simulink model "can_simple_block_bu11143"  (R2016b)
settings: Solver=FixedStepDiscrete  StartTime=0.0  StopTime=1000  FixedStep=0.2  RelTol=1e-3  EnableMultiTasking=on
undefined symbols (not defined in the file or in its folder): A, A10, A14, B, B11, B12, B13, B8, C, CS0, CS1, D, D11, D4, F3, F4, G, G3, G4, H3, H4, K17, K4, L3, N16, PA11, PA12, PD0, PE14, PE15, R10, R14, R17, SCK, SIN, SOUT, T14
libraries: rappid_564xl_ec_toolbox x59
(part 5 of 6)

== matlab function can_simple_block_bu11143/DataDumpFast1/RawData to StoreData15 ==
  data: StrCell input; CellV_1_104 data_store_memory; VTDataCAN_8b output uint8
function VTDataCAN_8b = fcn(StrCell)
global CellV_1_104;
onemask8 = uint16(hex2dec('00FF'));
onemask8_8sft = uint16(hex2dec('FF00'));
onemask8_56sft = uint64(hex2dec('FF'));
% yl = uint8(bitand(u,onemask8));
% yh = uint8(bitsra(bitand(u,onemask8_8sft),8));
% bitshift(remainder,8)  shift left
% bitsra(remainder,8)  shift right



VTDataCAN_8b =  uint8(zeros(1,8));
VTDataCAN_64b =  uint64(zeros(1,1));
VTDataCAN_4data =  uint8(zeros(1,4));

% VTDataCAN_4data(1) = fix(CellV_1_104(StrCell*4-3)/4);
% VTDataCAN_4data(2) = fix(CellV_1_104(StrCell*4-2)/4);
% VTDataCAN_4data(3) = fix(CellV_1_104(StrCell*4-1)/4);
% VTDataCAN_4data(4) = fix(CellV_1_104(StrCell*4-0)/4);

Bid = StrCell;
VTDataCAN_64b = uint64( Bid ) + ...
                            uint64( bitshift(uint64(CellV_1_104(StrCell*4-3)/4),8 ) ) + ...
                            uint64( bitshift(uint64(CellV_1_104(StrCell*4-2)/4),8+14 ))  + ...
                            uint64( bitshift(uint64(CellV_1_104(StrCell*4-1)/4),8+14+14)  )  + ...
                            uint64( bitshift(uint64(CellV_1_104(StrCell*4-0)/4),8+14+14+14) ) ;

VTDataCAN_8b(1) = uint8( bitand(VTDataCAN_64b,onemask8_56sft) );
VTDataCAN_8b(2) = uint8( bitand(bitsra(VTDataCAN_64b,8*1),onemask8_56sft) );
VTDataCAN_8b(3) = uint8( bitand(bitsra(VTDataCAN_64b,8*2),onemask8_56sft) );
VTDataCAN_8b(4) = uint8( bitand(bitsra(VTDataCAN_64b,8*3),onemask8_56sft) );
VTDataCAN_8b(5) = uint8( bitand(bitsra(VTDataCAN_64b,8*4),onemask8_56sft) );
VTDataCAN_8b(6) = uint8( bitand(bitsra(VTDataCAN_64b,8*5),onemask8_56sft) );
VTDataCAN_8b(7) = uint8( bitand(bitsra(VTDataCAN_64b,8*6),onemask8_56sft) );
VTDataCAN_8b(8) = uint8( bitand(bitsra(VTDataCAN_64b,8*7),onemask8_56sft) );

% VTDataCAN_8b(1) = Bid;
% VTDataCAN_8b(2) = VTDataCAN_4data(1)/(2^8);
% VTDataCAN_8b(3) = 4*fix(mod(CellV_1_104(StrCell*4-3),2^8)/4);
% VTDataCAN_8b(3) = VTDataCAN_8b(3) + CellV_1_104(StrCell*4-2)/(2^14);
% VTDataCAN_8b(4) = mod(CellV_1_104(StrCell*4-2),2^14) / (2^8);
% VTDataCAN_8b(5) =  * fix(mod(CellV_1_104(StrCell*4-2),2^6));

4*fix(CellV_1_104(StrCell*4-3)/4);


% VTDataCAN_8b(1) =         CellV_1_104(StrCell*4-3)/256;
% VTDataCAN_8b(2) = mod(CellV_1_104(StrCell*4-3),256);
% VTDataCAN_8b(3) =         CellV_1_104(StrCell*4-2)/256;
% VTDataCAN_8b(4) = mod(CellV_1_104(StrCell*4-2),256);
% VTDataCAN_8b(5) =         CellV_1_104(StrCell*4-1)/256;
% VTDataCAN_8b(6) = mod(CellV_1_104(StrCell*4-1),256);
% VTDataCAN_8b(7) =         CellV_1_104(StrCell*4   )/256;
% VTDataCAN_8b(8) = mod(CellV_1_104(StrCell*4   ),256);

% VTDataCAN_8b(1) =         CellV_1_104(1)/256;
% VTDataCAN_8b(2) = mod(CellV_1_104(1),256);
% VTDataCAN_8b(3) =         CellV_1_104(2)/256;
% VTDataCAN_8b(4) = mod(CellV_1_104(2),256);
% VTDataCAN_8b(5) =         CellV_1_104(9)/256;
% VTDataCAN_8b(6) = mod(CellV_1_104(9),256);
% VTDataCAN_8b(7) =         CellV_1_104(10)/256;
% VTDataCAN_8b(8) = mod(CellV_1_104(10),256);

% VTDataCAN_8b(1) =         uint16(30000)/256;
% VTDataCAN_8b(2) = mod(uint16(30000),256);
% VTDataCAN_8b(3) =         uint16(35000)/256;
% VTDataCAN_8b(4) = mod(uint16(35000),256);
% VTDataCAN_8b(5) =         uint16(33000)/256;
% VTDataCAN_8b(6) = mod(uint16(33000),256);
% VTDataCAN_8b(7) =         uint16(20000)/256;
% VTDataCAN_8b(8) = mod(uint16(20000),256);


end








% CellV_1_104(1) = uint16(1);

% SPIDataStore = uint16(zeros(1,21));
% DataFault =  zeros(1,7);
%
% for i=1:7
%   SPIDataStore(i*3-2) = SPIData(i*8-7)+SPIData(i*8-6)*256;
%   SPIDataStore(i*3-1) = SPIData(i*8-5)+SPIData(i*8-4)*256;
%   SPIDataStore(i*3   ) = SPIData(i*8-3)+SPIData(i*8-2)*256;
%   if (PecChk(i*2-1) == SPIData(i*8-1)) && (PecChk(i*2) == SPIData(i*8))
%     DataFault(i) = 1;
%   else
%     DataFault(i) = 0;
%   end
% end



% onemask8 = uint16(hex2dec('00FF'));
% onemask8_8sft = uint16(hex2dec('FF00'));
% onemask88 = uint8(hex2dec('FF'));
% onemask16 = uint16(hex2dec('FFFF'));
%
% % data_test = zeros(1,2);
% remainder = uint16(16);
%
% for i=1:len
%     ii = uint16(i);
% %     data_test(1,i) = data(ii);
% %     address = 2;
%     address = bitand( ...
%         bitxor( ...
%         uint8(bitsra(remainder,7)),data(ii) ), ...
%         onemask88);
%     remainder = bitxor(bitshift(remainder,8,'uint16'),pec15Table(address+1));
% end
% pec15 = uint16(bitand(bitshift(remainder,1,'uint16'),onemask16));
% pec0 = uint8(bitand(pec15,onemask8));
% pec1 = uint8(bitsra(bitand(pec15,onemask8_8sft),8));

== matlab function can_simple_block_bu11143/DataDumpFast1/RawData to StoreData16 ==
  data: StrCell input; CellV_1_104 data_store_memory; VTDataCAN_8b output uint8
function VTDataCAN_8b = fcn(StrCell)
global CellV_1_104;
onemask8 = uint16(hex2dec('00FF'));
onemask8_8sft = uint16(hex2dec('FF00'));
onemask8_56sft = uint64(hex2dec('FF'));
% yl = uint8(bitand(u,onemask8));
% yh = uint8(bitsra(bitand(u,onemask8_8sft),8));
% bitshift(remainder,8)  shift left
% bitsra(remainder,8)  shift right



VTDataCAN_8b =  uint8(zeros(1,8));
VTDataCAN_64b =  uint64(zeros(1,1));
VTDataCAN_4data =  uint8(zeros(1,4));

% VTDataCAN_4data(1) = fix(CellV_1_104(StrCell*4-3)/4);
% VTDataCAN_4data(2) = fix(CellV_1_104(StrCell*4-2)/4);
% VTDataCAN_4data(3) = fix(CellV_1_104(StrCell*4-1)/4);
% VTDataCAN_4data(4) = fix(CellV_1_104(StrCell*4-0)/4);

Bid = StrCell;
VTDataCAN_64b = uint64( Bid ) + ...
                            uint64( bitshift(uint64(CellV_1_104(StrCell*4-3)/4),8 ) ) + ...
                            uint64( bitshift(uint64(CellV_1_104(StrCell*4-2)/4),8+14 ))  + ...
                            uint64( bitshift(uint64(CellV_1_104(StrCell*4-1)/4),8+14+14)  )  + ...
                            uint64( bitshift(uint64(CellV_1_104(StrCell*4-0)/4),8+14+14+14) ) ;

VTDataCAN_8b(1) = uint8( bitand(VTDataCAN_64b,onemask8_56sft) );
VTDataCAN_8b(2) = uint8( bitand(bitsra(VTDataCAN_64b,8*1),onemask8_56sft) );
VTDataCAN_8b(3) = uint8( bitand(bitsra(VTDataCAN_64b,8*2),onemask8_56sft) );
VTDataCAN_8b(4) = uint8( bitand(bitsra(VTDataCAN_64b,8*3),onemask8_56sft) );
VTDataCAN_8b(5) = uint8( bitand(bitsra(VTDataCAN_64b,8*4),onemask8_56sft) );
VTDataCAN_8b(6) = uint8( bitand(bitsra(VTDataCAN_64b,8*5),onemask8_56sft) );
VTDataCAN_8b(7) = uint8( bitand(bitsra(VTDataCAN_64b,8*6),onemask8_56sft) );
VTDataCAN_8b(8) = uint8( bitand(bitsra(VTDataCAN_64b,8*7),onemask8_56sft) );

% VTDataCAN_8b(1) = Bid;
% VTDataCAN_8b(2) = VTDataCAN_4data(1)/(2^8);
% VTDataCAN_8b(3) = 4*fix(mod(CellV_1_104(StrCell*4-3),2^8)/4);
% VTDataCAN_8b(3) = VTDataCAN_8b(3) + CellV_1_104(StrCell*4-2)/(2^14);
% VTDataCAN_8b(4) = mod(CellV_1_104(StrCell*4-2),2^14) / (2^8);
% VTDataCAN_8b(5) =  * fix(mod(CellV_1_104(StrCell*4-2),2^6));

4*fix(CellV_1_104(StrCell*4-3)/4);


% VTDataCAN_8b(1) =         CellV_1_104(StrCell*4-3)/256;
% VTDataCAN_8b(2) = mod(CellV_1_104(StrCell*4-3),256);
% VTDataCAN_8b(3) =         CellV_1_104(StrCell*4-2)/256;
% VTDataCAN_8b(4) = mod(CellV_1_104(StrCell*4-2),256);
% VTDataCAN_8b(5) =         CellV_1_104(StrCell*4-1)/256;
% VTDataCAN_8b(6) = mod(CellV_1_104(StrCell*4-1),256);
% VTDataCAN_8b(7) =         CellV_1_104(StrCell*4   )/256;
% VTDataCAN_8b(8) = mod(CellV_1_104(StrCell*4   ),256);

% VTDataCAN_8b(1) =         CellV_1_104(1)/256;
% VTDataCAN_8b(2) = mod(CellV_1_104(1),256);
% VTDataCAN_8b(3) =         CellV_1_104(2)/256;
% VTDataCAN_8b(4) = mod(CellV_1_104(2),256);
% VTDataCAN_8b(5) =         CellV_1_104(9)/256;
% VTDataCAN_8b(6) = mod(CellV_1_104(9),256);
% VTDataCAN_8b(7) =         CellV_1_104(10)/256;
% VTDataCAN_8b(8) = mod(CellV_1_104(10),256);

% VTDataCAN_8b(1) =         uint16(30000)/256;
% VTDataCAN_8b(2) = mod(uint16(30000),256);
% VTDataCAN_8b(3) =         uint16(35000)/256;
% VTDataCAN_8b(4) = mod(uint16(35000),256);
% VTDataCAN_8b(5) =         uint16(33000)/256;
% VTDataCAN_8b(6) = mod(uint16(33000),256);
% VTDataCAN_8b(7) =         uint16(20000)/256;
% VTDataCAN_8b(8) = mod(uint16(20000),256);


end








% CellV_1_104(1) = uint16(1);

% SPIDataStore = uint16(zeros(1,21));
% DataFault =  zeros(1,7);
%
% for i=1:7
%   SPIDataStore(i*3-2) = SPIData(i*8-7)+SPIData(i*8-6)*256;
%   SPIDataStore(i*3-1) = SPIData(i*8-5)+SPIData(i*8-4)*256;
%   SPIDataStore(i*3   ) = SPIData(i*8-3)+SPIData(i*8-2)*256;
%   if (PecChk(i*2-1) == SPIData(i*8-1)) && (PecChk(i*2) == SPIData(i*8))
%     DataFault(i) = 1;
%   else
%     DataFault(i) = 0;
%   end
% end



% onemask8 = uint16(hex2dec('00FF'));
% onemask8_8sft = uint16(hex2dec('FF00'));
% onemask88 = uint8(hex2dec('FF'));
% onemask16 = uint16(hex2dec('FFFF'));
%
% % data_test = zeros(1,2);
% remainder = uint16(16);
%
% for i=1:len
%     ii = uint16(i);
% %     data_test(1,i) = data(ii);
% %     address = 2;
%     address = bitand( ...
%         bitxor( ...
%         uint8(bitsra(remainder,7)),data(ii) ), ...
%         onemask88);
%     remainder = bitxor(bitshift(remainder,8,'uint16'),pec15Table(address+1));
% end
% pec15 = uint16(bitand(bitshift(remainder,1,'uint16'),onemask16));
% pec0 = uint8(bitand(pec15,onemask8));
% pec1 = uint8(bitsra(bitand(pec15,onemask8_8sft),8));

== stateflow chart can_simple_block_bu11143/DataDumpFast/Chart2 ==
  state A
    en: count  = count + 1;
    du: count = count + 1;
  state A1
    en: count = 1;
  (default) -> A : {count =0;}
  A1 -> A
  A -> A1 : [count >= count_in]
  data: count_in input; count output double [0..10000]

== matlab function can_simple_block_bu11143/DataDumpFast/RawData to StoreData1 ==
  data: StrCell input; CellGP_1_78 data_store_memory; VTDataCAN_8b output uint8
function VTDataCAN_8b = fcn(StrCell)

% global CellV_1_104;
global CellGP_1_78;
VTDataCAN_8b =  uint8(zeros(1,8));
% 
% StrCell_2 = fix((StrCell+1)/2);
% 
% if mod(StrCell,2)==1
% VTDataCAN_8b(1) =         CellGP_1_78(StrCell_2*6-5)/256;
% VTDataCAN_8b(2) = mod(CellGP_1_78(StrCell_2*6-5),256);
% VTDataCAN_8b(3) =         CellGP_1_78(StrCell_2*6-4)/256;
% VTDataCAN_8b(4) = mod(CellGP_1_78(StrCell_2*6-4),256);
% VTDataCAN_8b(5) =         CellGP_1_78(StrCell_2*6-3)/256;
% VTDataCAN_8b(6) = mod(CellGP_1_78(StrCell_2*6-3),256);
% VTDataCAN_8b(7) =         CellGP_1_78(StrCell_2*6-2 )/256;
% VTDataCAN_8b(8) = mod(CellGP_1_78(StrCell_2*6-2),256);
% else 
% VTDataCAN_8b(1) =         CellGP_1_78(StrCell_2*6-1 )/256;
% VTDataCAN_8b(2) = mod(CellGP_1_78(StrCell_2*6-1 ),256);
% VTDataCAN_8b(3) =         CellGP_1_78(StrCell_2*6-0 )/256;
% VTDataCAN_8b(4) = mod(CellGP_1_78(StrCell_2*6-0 ),256);
% end
onemask8 = uint16(hex2dec('00FF'));
onemask8_8sft = uint16(hex2dec('FF00'));
onemask8_56sft = uint64(hex2dec('FF'));
VTDataCAN_8b =  uint8(zeros(1,8));
VTDataCAN_64b =  uint64(zeros(1,1));
VTDataCAN_4data =  uint8(zeros(1,4));

Bid = StrCell;
VTDataCAN_64b = uint64( Bid ) + ...
                            uint64( bitshift(uint64(CellGP_1_78(StrCell*6-5)/64),8 ) ) + ...
                            uint64( bitshift(uint64(CellGP_1_78(StrCell*6-4)/64),8+10*1 ) )  + ...
                            uint64( bitshift(uint64(CellGP_1_78(StrCell*6-3)/64),8+10*2 ) )  + ...
                            uint64( bitshift(uint64(CellGP_1_78(StrCell*6-2)/64),8+10*3 ) ) + ...
                            uint64( bitshift(uint64(CellGP_1_78(StrCell*6-1)/64),8+10*4 ) ) + ...
                            uint64( bitshift(uint64(CellGP_1_78(StrCell*6-0)/1024),8+10*5 ) ) ;

VTDataCAN_8b(1) = uint8( bitand(VTDataCAN_64b,onemask8_56sft) );
VTDataCAN_8b(2) = uint8( bitand(bitsra(VTDataCAN_64b,8*1),onemask8_56sft) );
VTDataCAN_8b(3) = uint8( bitand(bitsra(VTDataCAN_64b,8*2),onemask8_56sft) );
VTDataCAN_8b(4) = uint8( bitand(bitsra(VTDataCAN_64b,8*3),onemask8_56sft) );
VTDataCAN_8b(5) = uint8( bitand(bitsra(VTDataCAN_64b,8*4),onemask8_56sft) );
VTDataCAN_8b(6) = uint8( bitand(bitsra(VTDataCAN_64b,8*5),onemask8_56sft) );
VTDataCAN_8b(7) = uint8( bitand(bitsra(VTDataCAN_64b,8*6),onemask8_56sft) );
VTDataCAN_8b(8) = uint8( bitand(bitsra(VTDataCAN_64b,8*7),onemask8_56sft) );


% VTDataCAN_8b(1) =         CellV_1_104(1)/256;
% VTDataCAN_8b(2) = mod(CellV_1_104(1),256);
% VTDataCAN_8b(3) =         CellV_1_104(2)/256;
% VTDataCAN_8b(4) = mod(CellV_1_104(2),256);
% VTDataCAN_8b(5) =         CellV_1_104(9)/256;
% VTDataCAN_8b(6) = mod(CellV_1_104(9),256);
% VTDataCAN_8b(7) =         CellV_1_104(10)/256;
% VTDataCAN_8b(8) = mod(CellV_1_104(10),256);

% VTDataCAN_8b(1) =         uint16(30000)/256;
% VTDataCAN_8b(2) = mod(uint16(30000),256);
% VTDataCAN_8b(3) =         uint16(35000)/256;
% VTDataCAN_8b(4) = mod(uint16(35000),256);
% VTDataCAN_8b(5) =         uint16(33000)/256;
% VTDataCAN_8b(6) = mod(uint16(33000),256);
% VTDataCAN_8b(7) =         uint16(20000)/256;
% VTDataCAN_8b(8) = mod(uint16(20000),256);


end








% CellV_1_104(1) = uint16(1);

% SPIDataStore = uint16(zeros(1,21));
% DataFault =  zeros(1,7);
%
% for i=1:7
%   SPIDataStore(i*3-2) = SPIData(i*8-7)+SPIData(i*8-6)*256;
%   SPIDataStore(i*3-1) = SPIData(i*8-5)+SPIData(i*8-4)*256;
%   SPIDataStore(i*3   ) = SPIData(i*8-3)+SPIData(i*8-2)*256;
%   if (PecChk(i*2-1) == SPIData(i*8-1)) && (PecChk(i*2) == SPIData(i*8))
%     DataFault(i) = 1;
%   else
%     DataFault(i) = 0;
%   end
% end



% onemask8 = uint16(hex2dec('00FF'));
% onemask8_8sft = uint16(hex2dec('FF00'));
% onemask88 = uint8(hex2dec('FF'));
% onemask16 = uint16(hex2dec('FFFF'));
%
% % data_test = zeros(1,2);
% remainder = uint16(16);
%
% for i=1:len
%     ii = uint16(i);
% %     data_test(1,i) = data(ii);
% %     address = 2;
%     address = bitand( ...
%         bitxor( ...
%         uint8(bitsra(remainder,7)),data(ii) ), ...
%         onemask88);
%     remainder = bitxor(bitshift(remainder,8,'uint16'),pec15Table(address+1));
% end
% pec15 = uint16(bitand(bitshift(remainder,1,'uint16'),onemask16));
% pec0 = uint8(bitand(pec15,onemask8));
% pec1 = uint8(bitsra(bitand(pec15,onemask8_8sft),8));

== matlab function can_simple_block_bu11143/DataDumpFast1/RawData to StoreData17 ==
  data: StrCell input; CellV_1_104 data_store_memory; VTDataCAN_8b output uint8
function VTDataCAN_8b = fcn(StrCell)
global CellV_1_104;
onemask8 = uint16(hex2dec('00FF'));
onemask8_8sft = uint16(hex2dec('FF00'));
onemask8_56sft = uint64(hex2dec('FF'));
% yl = uint8(bitand(u,onemask8));
% yh = uint8(bitsra(bitand(u,onemask8_8sft),8));
% bitshift(remainder,8)  shift left
% bitsra(remainder,8)  shift right



VTDataCAN_8b =  uint8(zeros(1,8));
VTDataCAN_64b =  uint64(zeros(1,1));
VTDataCAN_4data =  uint8(zeros(1,4));

% VTDataCAN_4data(1) = fix(CellV_1_104(StrCell*4-3)/4);
% VTDataCAN_4data(2) = fix(CellV_1_104(StrCell*4-2)/4);
% VTDataCAN_4data(3) = fix(CellV_1_104(StrCell*4-1)/4);
% VTDataCAN_4data(4) = fix(CellV_1_104(StrCell*4-0)/4);

Bid = StrCell;
VTDataCAN_64b = uint64( Bid ) + ...
                            uint64( bitshift(uint64(CellV_1_104(StrCell*4-3)/4),8 ) ) + ...
                            uint64( bitshift(uint64(CellV_1_104(StrCell*4-2)/4),8+14 ))  + ...
                            uint64( bitshift(uint64(CellV_1_104(StrCell*4-1)/4),8+14+14)  )  + ...
                            uint64( bitshift(uint64(CellV_1_104(StrCell*4-0)/4),8+14+14+14) ) ;

VTDataCAN_8b(1) = uint8( bitand(VTDataCAN_64b,onemask8_56sft) );
VTDataCAN_8b(2) = uint8( bitand(bitsra(VTDataCAN_64b,8*1),onemask8_56sft) );
VTDataCAN_8b(3) = uint8( bitand(bitsra(VTDataCAN_64b,8*2),onemask8_56sft) );
VTDataCAN_8b(4) = uint8( bitand(bitsra(VTDataCAN_64b,8*3),onemask8_56sft) );
VTDataCAN_8b(5) = uint8( bitand(bitsra(VTDataCAN_64b,8*4),onemask8_56sft) );
VTDataCAN_8b(6) = uint8( bitand(bitsra(VTDataCAN_64b,8*5),onemask8_56sft) );
VTDataCAN_8b(7) = uint8( bitand(bitsra(VTDataCAN_64b,8*6),onemask8_56sft) );
VTDataCAN_8b(8) = uint8( bitand(bitsra(VTDataCAN_64b,8*7),onemask8_56sft) );

% VTDataCAN_8b(1) = Bid;
% VTDataCAN_8b(2) = VTDataCAN_4data(1)/(2^8);
% VTDataCAN_8b(3) = 4*fix(mod(CellV_1_104(StrCell*4-3),2^8)/4);
% VTDataCAN_8b(3) = VTDataCAN_8b(3) + CellV_1_104(StrCell*4-2)/(2^14);
% VTDataCAN_8b(4) = mod(CellV_1_104(StrCell*4-2),2^14) / (2^8);
% VTDataCAN_8b(5) =  * fix(mod(CellV_1_104(StrCell*4-2),2^6));

4*fix(CellV_1_104(StrCell*4-3)/4);


% VTDataCAN_8b(1) =         CellV_1_104(StrCell*4-3)/256;
% VTDataCAN_8b(2) = mod(CellV_1_104(StrCell*4-3),256);
% VTDataCAN_8b(3) =         CellV_1_104(StrCell*4-2)/256;
% VTDataCAN_8b(4) = mod(CellV_1_104(StrCell*4-2),256);
% VTDataCAN_8b(5) =         CellV_1_104(StrCell*4-1)/256;
% VTDataCAN_8b(6) = mod(CellV_1_104(StrCell*4-1),256);
% VTDataCAN_8b(7) =         CellV_1_104(StrCell*4   )/256;
% VTDataCAN_8b(8) = mod(CellV_1_104(StrCell*4   ),256);

% VTDataCAN_8b(1) =         CellV_1_104(1)/256;
% VTDataCAN_8b(2) = mod(CellV_1_104(1),256);
% VTDataCAN_8b(3) =         CellV_1_104(2)/256;
% VTDataCAN_8b(4) = mod(CellV_1_104(2),256);
% VTDataCAN_8b(5) =         CellV_1_104(9)/256;
% VTDataCAN_8b(6) = mod(CellV_1_104(9),256);
% VTDataCAN_8b(7) =         CellV_1_104(10)/256;
% VTDataCAN_8b(8) = mod(CellV_1_104(10),256);

% VTDataCAN_8b(1) =         uint16(30000)/256;
% VTDataCAN_8b(2) = mod(uint16(30000),256);
% VTDataCAN_8b(3) =         uint16(35000)/256;
% VTDataCAN_8b(4) = mod(uint16(35000),256);
% VTDataCAN_8b(5) =         uint16(33000)/256;
% VTDataCAN_8b(6) = mod(uint16(33000),256);
% VTDataCAN_8b(7) =         uint16(20000)/256;
% VTDataCAN_8b(8) = mod(uint16(20000),256);


end








% CellV_1_104(1) = uint16(1);

% SPIDataStore = uint16(zeros(1,21));
% DataFault =  zeros(1,7);
%
% for i=1:7
%   SPIDataStore(i*3-2) = SPIData(i*8-7)+SPIData(i*8-6)*256;
%   SPIDataStore(i*3-1) = SPIData(i*8-5)+SPIData(i*8-4)*256;
%   SPIDataStore(i*3   ) = SPIData(i*8-3)+SPIData(i*8-2)*256;
%   if (PecChk(i*2-1) == SPIData(i*8-1)) && (PecChk(i*2) == SPIData(i*8))
%     DataFault(i) = 1;
%   else
%     DataFault(i) = 0;
%   end
% end



% onemask8 = uint16(hex2dec('00FF'));
% onemask8_8sft = uint16(hex2dec('FF00'));
% onemask88 = uint8(hex2dec('FF'));
% onemask16 = uint16(hex2dec('FFFF'));
%
% % data_test = zeros(1,2);
% remainder = uint16(16);
%
% for i=1:len
%     ii = uint16(i);
% %     data_test(1,i) = data(ii);
% %     address = 2;
%     address = bitand( ...
%         bitxor( ...
%         uint8(bitsra(remainder,7)),data(ii) ), ...
%         onemask88);
%     remainder = bitxor(bitshift(remainder,8,'uint16'),pec15Table(address+1));
% end
% pec15 = uint16(bitand(bitshift(remainder,1,'uint16'),onemask16));
% pec0 = uint8(bitand(pec15,onemask8));
% pec1 = uint8(bitsra(bitand(pec15,onemask8_8sft),8));

== matlab function can_simple_block_bu11143/DataDumpFast1/RawData to StoreData18 ==
  data: StrCell input; CellV_1_104 data_store_memory; VTDataCAN_8b output uint8
function VTDataCAN_8b = fcn(StrCell)
global CellV_1_104;
onemask8 = uint16(hex2dec('00FF'));
onemask8_8sft = uint16(hex2dec('FF00'));
onemask8_56sft = uint64(hex2dec('FF'));
% yl = uint8(bitand(u,onemask8));
% yh = uint8(bitsra(bitand(u,onemask8_8sft),8));
% bitshift(remainder,8)  shift left
% bitsra(remainder,8)  shift right



VTDataCAN_8b =  uint8(zeros(1,8));
VTDataCAN_64b =  uint64(zeros(1,1));
VTDataCAN_4data =  uint8(zeros(1,4));

% VTDataCAN_4data(1) = fix(CellV_1_104(StrCell*4-3)/4);
% VTDataCAN_4data(2) = fix(CellV_1_104(StrCell*4-2)/4);
% VTDataCAN_4data(3) = fix(CellV_1_104(StrCell*4-1)/4);
% VTDataCAN_4data(4) = fix(CellV_1_104(StrCell*4-0)/4);

Bid = StrCell;
VTDataCAN_64b = uint64( Bid ) + ...
                            uint64( bitshift(uint64(CellV_1_104(StrCell*4-3)/4),8 ) ) + ...
                            uint64( bitshift(uint64(CellV_1_104(StrCell*4-2)/4),8+14 ))  + ...
                            uint64( bitshift(uint64(CellV_1_104(StrCell*4-1)/4),8+14+14)  )  + ...
                            uint64( bitshift(uint64(CellV_1_104(StrCell*4-0)/4),8+14+14+14) ) ;

VTDataCAN_8b(1) = uint8( bitand(VTDataCAN_64b,onemask8_56sft) );
VTDataCAN_8b(2) = uint8( bitand(bitsra(VTDataCAN_64b,8*1),onemask8_56sft) );
VTDataCAN_8b(3) = uint8( bitand(bitsra(VTDataCAN_64b,8*2),onemask8_56sft) );
VTDataCAN_8b(4) = uint8( bitand(bitsra(VTDataCAN_64b,8*3),onemask8_56sft) );
VTDataCAN_8b(5) = uint8( bitand(bitsra(VTDataCAN_64b,8*4),onemask8_56sft) );
VTDataCAN_8b(6) = uint8( bitand(bitsra(VTDataCAN_64b,8*5),onemask8_56sft) );
VTDataCAN_8b(7) = uint8( bitand(bitsra(VTDataCAN_64b,8*6),onemask8_56sft) );
VTDataCAN_8b(8) = uint8( bitand(bitsra(VTDataCAN_64b,8*7),onemask8_56sft) );

% VTDataCAN_8b(1) = Bid;
% VTDataCAN_8b(2) = VTDataCAN_4data(1)/(2^8);
% VTDataCAN_8b(3) = 4*fix(mod(CellV_1_104(StrCell*4-3),2^8)/4);
% VTDataCAN_8b(3) = VTDataCAN_8b(3) + CellV_1_104(StrCell*4-2)/(2^14);
% VTDataCAN_8b(4) = mod(CellV_1_104(StrCell*4-2),2^14) / (2^8);
% VTDataCAN_8b(5) =  * fix(mod(CellV_1_104(StrCell*4-2),2^6));

4*fix(CellV_1_104(StrCell*4-3)/4);


% VTDataCAN_8b(1) =         CellV_1_104(StrCell*4-3)/256;
% VTDataCAN_8b(2) = mod(CellV_1_104(StrCell*4-3),256);
% VTDataCAN_8b(3) =         CellV_1_104(StrCell*4-2)/256;
% VTDataCAN_8b(4) = mod(CellV_1_104(StrCell*4-2),256);
% VTDataCAN_8b(5) =         CellV_1_104(StrCell*4-1)/256;
% VTDataCAN_8b(6) = mod(CellV_1_104(StrCell*4-1),256);
% VTDataCAN_8b(7) =         CellV_1_104(StrCell*4   )/256;
% VTDataCAN_8b(8) = mod(CellV_1_104(StrCell*4   ),256);

% VTDataCAN_8b(1) =         CellV_1_104(1)/256;
% VTDataCAN_8b(2) = mod(CellV_1_104(1),256);
% VTDataCAN_8b(3) =         CellV_1_104(2)/256;
% VTDataCAN_8b(4) = mod(CellV_1_104(2),256);
% VTDataCAN_8b(5) =         CellV_1_104(9)/256;
% VTDataCAN_8b(6) = mod(CellV_1_104(9),256);
% VTDataCAN_8b(7) =         CellV_1_104(10)/256;
% VTDataCAN_8b(8) = mod(CellV_1_104(10),256);

% VTDataCAN_8b(1) =         uint16(30000)/256;
% VTDataCAN_8b(2) = mod(uint16(30000),256);
% VTDataCAN_8b(3) =         uint16(35000)/256;
% VTDataCAN_8b(4) = mod(uint16(35000),256);
% VTDataCAN_8b(5) =         uint16(33000)/256;
% VTDataCAN_8b(6) = mod(uint16(33000),256);
% VTDataCAN_8b(7) =         uint16(20000)/256;
% VTDataCAN_8b(8) = mod(uint16(20000),256);


end








% CellV_1_104(1) = uint16(1);

% SPIDataStore = uint16(zeros(1,21));
% DataFault =  zeros(1,7);
%
% for i=1:7
%   SPIDataStore(i*3-2) = SPIData(i*8-7)+SPIData(i*8-6)*256;
%   SPIDataStore(i*3-1) = SPIData(i*8-5)+SPIData(i*8-4)*256;
%   SPIDataStore(i*3   ) = SPIData(i*8-3)+SPIData(i*8-2)*256;
%   if (PecChk(i*2-1) == SPIData(i*8-1)) && (PecChk(i*2) == SPIData(i*8))
%     DataFault(i) = 1;
%   else
%     DataFault(i) = 0;
%   end
% end



% onemask8 = uint16(hex2dec('00FF'));
% onemask8_8sft = uint16(hex2dec('FF00'));
% onemask88 = uint8(hex2dec('FF'));
% onemask16 = uint16(hex2dec('FFFF'));
%
% % data_test = zeros(1,2);
% remainder = uint16(16);
%
% for i=1:len
%     ii = uint16(i);
% %     data_test(1,i) = data(ii);
% %     address = 2;
%     address = bitand( ...
%         bitxor( ...
%         uint8(bitsra(remainder,7)),data(ii) ), ...
%         onemask88);
%     remainder = bitxor(bitshift(remainder,8,'uint16'),pec15Table(address+1));
% end
% pec15 = uint16(bitand(bitshift(remainder,1,'uint16'),onemask16));
% pec0 = uint8(bitand(pec15,onemask8));
% pec1 = uint8(bitsra(bitand(pec15,onemask8_8sft),8));

== matlab function can_simple_block_bu11143/DataDumpFast1/RawData to StoreData19 ==
  data: StrCell input; CellV_1_104 data_store_memory; VTDataCAN_8b output uint8
function VTDataCAN_8b = fcn(StrCell)
global CellV_1_104;
onemask8 = uint16(hex2dec('00FF'));
onemask8_8sft = uint16(hex2dec('FF00'));
onemask8_56sft = uint64(hex2dec('FF'));
% yl = uint8(bitand(u,onemask8));
% yh = uint8(bitsra(bitand(u,onemask8_8sft),8));
% bitshift(remainder,8)  shift left
% bitsra(remainder,8)  shift right



VTDataCAN_8b =  uint8(zeros(1,8));
VTDataCAN_64b =  uint64(zeros(1,1));
VTDataCAN_4data =  uint8(zeros(1,4));

% VTDataCAN_4data(1) = fix(CellV_1_104(StrCell*4-3)/4);
% VTDataCAN_4data(2) = fix(CellV_1_104(StrCell*4-2)/4);
% VTDataCAN_4data(3) = fix(CellV_1_104(StrCell*4-1)/4);
% VTDataCAN_4data(4) = fix(CellV_1_104(StrCell*4-0)/4);

Bid = StrCell;
VTDataCAN_64b = uint64( Bid ) + ...
                            uint64( bitshift(uint64(CellV_1_104(StrCell*4-3)/4),8 ) ) + ...
                            uint64( bitshift(uint64(CellV_1_104(StrCell*4-2)/4),8+14 ))  + ...
                            uint64( bitshift(uint64(CellV_1_104(StrCell*4-1)/4),8+14+14)  )  + ...
                            uint64( bitshift(uint64(CellV_1_104(StrCell*4-0)/4),8+14+14+14) ) ;

VTDataCAN_8b(1) = uint8( bitand(VTDataCAN_64b,onemask8_56sft) );
VTDataCAN_8b(2) = uint8( bitand(bitsra(VTDataCAN_64b,8*1),onemask8_56sft) );
VTDataCAN_8b(3) = uint8( bitand(bitsra(VTDataCAN_64b,8*2),onemask8_56sft) );
VTDataCAN_8b(4) = uint8( bitand(bitsra(VTDataCAN_64b,8*3),onemask8_56sft) );
VTDataCAN_8b(5) = uint8( bitand(bitsra(VTDataCAN_64b,8*4),onemask8_56sft) );
VTDataCAN_8b(6) = uint8( bitand(bitsra(VTDataCAN_64b,8*5),onemask8_56sft) );
VTDataCAN_8b(7) = uint8( bitand(bitsra(VTDataCAN_64b,8*6),onemask8_56sft) );
VTDataCAN_8b(8) = uint8( bitand(bitsra(VTDataCAN_64b,8*7),onemask8_56sft) );

% VTDataCAN_8b(1) = Bid;
% VTDataCAN_8b(2) = VTDataCAN_4data(1)/(2^8);
% VTDataCAN_8b(3) = 4*fix(mod(CellV_1_104(StrCell*4-3),2^8)/4);
% VTDataCAN_8b(3) = VTDataCAN_8b(3) + CellV_1_104(StrCell*4-2)/(2^14);
% VTDataCAN_8b(4) = mod(CellV_1_104(StrCell*4-2),2^14) / (2^8);
% VTDataCAN_8b(5) =  * fix(mod(CellV_1_104(StrCell*4-2),2^6));

4*fix(CellV_1_104(StrCell*4-3)/4);


% VTDataCAN_8b(1) =         CellV_1_104(StrCell*4-3)/256;
% VTDataCAN_8b(2) = mod(CellV_1_104(StrCell*4-3),256);
% VTDataCAN_8b(3) =         CellV_1_104(StrCell*4-2)/256;
% VTDataCAN_8b(4) = mod(CellV_1_104(StrCell*4-2),256);
% VTDataCAN_8b(5) =         CellV_1_104(StrCell*4-1)/256;
% VTDataCAN_8b(6) = mod(CellV_1_104(StrCell*4-1),256);
% VTDataCAN_8b(7) =         CellV_1_104(StrCell*4   )/256;
% VTDataCAN_8b(8) = mod(CellV_1_104(StrCell*4   ),256);

% VTDataCAN_8b(1) =         CellV_1_104(1)/256;
% VTDataCAN_8b(2) = mod(CellV_1_104(1),256);
% VTDataCAN_8b(3) =         CellV_1_104(2)/256;
% VTDataCAN_8b(4) = mod(CellV_1_104(2),256);
% VTDataCAN_8b(5) =         CellV_1_104(9)/256;
% VTDataCAN_8b(6) = mod(CellV_1_104(9),256);
% VTDataCAN_8b(7) =         CellV_1_104(10)/256;
% VTDataCAN_8b(8) = mod(CellV_1_104(10),256);

% VTDataCAN_8b(1) =         uint16(30000)/256;
% VTDataCAN_8b(2) = mod(uint16(30000),256);
% VTDataCAN_8b(3) =         uint16(35000)/256;
% VTDataCAN_8b(4) = mod(uint16(35000),256);
% VTDataCAN_8b(5) =         uint16(33000)/256;
% VTDataCAN_8b(6) = mod(uint16(33000),256);
% VTDataCAN_8b(7) =         uint16(20000)/256;
% VTDataCAN_8b(8) = mod(uint16(20000),256);


end








% CellV_1_104(1) = uint16(1);

% SPIDataStore = uint16(zeros(1,21));
% DataFault =  zeros(1,7);
%
% for i=1:7
%   SPIDataStore(i*3-2) = SPIData(i*8-7)+SPIData(i*8-6)*256;
%   SPIDataStore(i*3-1) = SPIData(i*8-5)+SPIData(i*8-4)*256;
%   SPIDataStore(i*3   ) = SPIData(i*8-3)+SPIData(i*8-2)*256;
%   if (PecChk(i*2-1) == SPIData(i*8-1)) && (PecChk(i*2) == SPIData(i*8))
%     DataFault(i) = 1;
%   else
%     DataFault(i) = 0;
%   end
% end



% onemask8 = uint16(hex2dec('00FF'));
% onemask8_8sft = uint16(hex2dec('FF00'));
% onemask88 = uint8(hex2dec('FF'));
% onemask16 = uint16(hex2dec('FFFF'));
%
% % data_test = zeros(1,2);
% remainder = uint16(16);
%
% for i=1:len
%     ii = uint16(i);
% %     data_test(1,i) = data(ii);
% %     address = 2;
%     address = bitand( ...
%         bitxor( ...
%         uint8(bitsra(remainder,7)),data(ii) ), ...
%         onemask88);
%     remainder = bitxor(bitshift(remainder,8,'uint16'),pec15Table(address+1));
% end
% pec15 = uint16(bitand(bitshift(remainder,1,'uint16'),onemask16));
% pec0 = uint8(bitand(pec15,onemask8));
% pec1 = uint8(bitsra(bitand(pec15,onemask8_8sft),8));

== matlab function can_simple_block_bu11143/DataDumpFast1/RawData to StoreData20 ==
  data: StrCell input; CellV_1_104 data_store_memory; VTDataCAN_8b output uint8
function VTDataCAN_8b = fcn(StrCell)
global CellV_1_104;
onemask8 = uint16(hex2dec('00FF'));
onemask8_8sft = uint16(hex2dec('FF00'));
onemask8_56sft = uint64(hex2dec('FF'));
% yl = uint8(bitand(u,onemask8));
% yh = uint8(bitsra(bitand(u,onemask8_8sft),8));
% bitshift(remainder,8)  shift left
% bitsra(remainder,8)  shift right



VTDataCAN_8b =  uint8(zeros(1,8));
VTDataCAN_64b =  uint64(zeros(1,1));
VTDataCAN_4data =  uint8(zeros(1,4));

% VTDataCAN_4data(1) = fix(CellV_1_104(StrCell*4-3)/4);
% VTDataCAN_4data(2) = fix(CellV_1_104(StrCell*4-2)/4);
% VTDataCAN_4data(3) = fix(CellV_1_104(StrCell*4-1)/4);
% VTDataCAN_4data(4) = fix(CellV_1_104(StrCell*4-0)/4);

Bid = StrCell;
VTDataCAN_64b = uint64( Bid ) + ...
                            uint64( bitshift(uint64(CellV_1_104(StrCell*4-3)/4),8 ) ) + ...
                            uint64( bitshift(uint64(CellV_1_104(StrCell*4-2)/4),8+14 ))  + ...
                            uint64( bitshift(uint64(CellV_1_104(StrCell*4-1)/4),8+14+14)  )  + ...
                            uint64( bitshift(uint64(CellV_1_104(StrCell*4-0)/4),8+14+14+14) ) ;

VTDataCAN_8b(1) = uint8( bitand(VTDataCAN_64b,onemask8_56sft) );
VTDataCAN_8b(2) = uint8( bitand(bitsra(VTDataCAN_64b,8*1),onemask8_56sft) );
VTDataCAN_8b(3) = uint8( bitand(bitsra(VTDataCAN_64b,8*2),onemask8_56sft) );
VTDataCAN_8b(4) = uint8( bitand(bitsra(VTDataCAN_64b,8*3),onemask8_56sft) );
VTDataCAN_8b(5) = uint8( bitand(bitsra(VTDataCAN_64b,8*4),onemask8_56sft) );
VTDataCAN_8b(6) = uint8( bitand(bitsra(VTDataCAN_64b,8*5),onemask8_56sft) );
VTDataCAN_8b(7) = uint8( bitand(bitsra(VTDataCAN_64b,8*6),onemask8_56sft) );
VTDataCAN_8b(8) = uint8( bitand(bitsra(VTDataCAN_64b,8*7),onemask8_56sft) );

% VTDataCAN_8b(1) = Bid;
% VTDataCAN_8b(2) = VTDataCAN_4data(1)/(2^8);
% VTDataCAN_8b(3) = 4*fix(mod(CellV_1_104(StrCell*4-3),2^8)/4);
% VTDataCAN_8b(3) = VTDataCAN_8b(3) + CellV_1_104(StrCell*4-2)/(2^14);
% VTDataCAN_8b(4) = mod(CellV_1_104(StrCell*4-2),2^14) / (2^8);
% VTDataCAN_8b(5) =  * fix(mod(CellV_1_104(StrCell*4-2),2^6));

4*fix(CellV_1_104(StrCell*4-3)/4);


% VTDataCAN_8b(1) =         CellV_1_104(StrCell*4-3)/256;
% VTDataCAN_8b(2) = mod(CellV_1_104(StrCell*4-3),256);
% VTDataCAN_8b(3) =         CellV_1_104(StrCell*4-2)/256;
% VTDataCAN_8b(4) = mod(CellV_1_104(StrCell*4-2),256);
% VTDataCAN_8b(5) =         CellV_1_104(StrCell*4-1)/256;
% VTDataCAN_8b(6) = mod(CellV_1_104(StrCell*4-1),256);
% VTDataCAN_8b(7) =         CellV_1_104(StrCell*4   )/256;
% VTDataCAN_8b(8) = mod(CellV_1_104(StrCell*4   ),256);

% VTDataCAN_8b(1) =         CellV_1_104(1)/256;
% VTDataCAN_8b(2) = mod(CellV_1_104(1),256);
% VTDataCAN_8b(3) =         CellV_1_104(2)/256;
% VTDataCAN_8b(4) = mod(CellV_1_104(2),256);
% VTDataCAN_8b(5) =         CellV_1_104(9)/256;
% VTDataCAN_8b(6) = mod(CellV_1_104(9),256);
% VTDataCAN_8b(7) =         CellV_1_104(10)/256;
% VTDataCAN_8b(8) = mod(CellV_1_104(10),256);

% VTDataCAN_8b(1) =         uint16(30000)/256;
% VTDataCAN_8b(2) = mod(uint16(30000),256);
% VTDataCAN_8b(3) =         uint16(35000)/256;
% VTDataCAN_8b(4) = mod(uint16(35000),256);
% VTDataCAN_8b(5) =         uint16(33000)/256;
% VTDataCAN_8b(6) = mod(uint16(33000),256);
% VTDataCAN_8b(7) =         uint16(20000)/256;
% VTDataCAN_8b(8) = mod(uint16(20000),256);


end








% CellV_1_104(1) = uint16(1);

% SPIDataStore = uint16(zeros(1,21));
% DataFault =  zeros(1,7);
%
% for i=1:7
%   SPIDataStore(i*3-2) = SPIData(i*8-7)+SPIData(i*8-6)*256;
%   SPIDataStore(i*3-1) = SPIData(i*8-5)+SPIData(i*8-4)*256;
%   SPIDataStore(i*3   ) = SPIData(i*8-3)+SPIData(i*8-2)*256;
%   if (PecChk(i*2-1) == SPIData(i*8-1)) && (PecChk(i*2) == SPIData(i*8))
%     DataFault(i) = 1;
%   else
%     DataFault(i) = 0;
%   end
% end



% onemask8 = uint16(hex2dec('00FF'));
% onemask8_8sft = uint16(hex2dec('FF00'));
% onemask88 = uint8(hex2dec('FF'));
% onemask16 = uint16(hex2dec('FFFF'));
%
% % data_test = zeros(1,2);
% remainder = uint16(16);
%
% for i=1:len
%     ii = uint16(i);
% %     data_test(1,i) = data(ii);
% %     address = 2;
%     address = bitand( ...
%         bitxor( ...
%         uint8(bitsra(remainder,7)),data(ii) ), ...
%         onemask88);
%     remainder = bitxor(bitshift(remainder,8,'uint16'),pec15Table(address+1));
% end
% pec15 = uint16(bitand(bitshift(remainder,1,'uint16'),onemask16));
% pec0 = uint8(bitand(pec15,onemask8));
% pec1 = uint8(bitsra(bitand(pec15,onemask8_8sft),8));

== matlab function can_simple_block_bu11143/DataDumpFast1/RawData to StoreData21 ==
  data: StrCell input; CellV_1_104 data_store_memory; VTDataCAN_8b output uint8
function VTDataCAN_8b = fcn(StrCell)
global CellV_1_104;
onemask8 = uint16(hex2dec('00FF'));
onemask8_8sft = uint16(hex2dec('FF00'));
onemask8_56sft = uint64(hex2dec('FF'));
% yl = uint8(bitand(u,onemask8));
% yh = uint8(bitsra(bitand(u,onemask8_8sft),8));
% bitshift(remainder,8)  shift left
% bitsra(remainder,8)  shift right



VTDataCAN_8b =  uint8(zeros(1,8));
VTDataCAN_64b =  uint64(zeros(1,1));
VTDataCAN_4data =  uint8(zeros(1,4));

% VTDataCAN_4data(1) = fix(CellV_1_104(StrCell*4-3)/4);
% VTDataCAN_4data(2) = fix(CellV_1_104(StrCell*4-2)/4);
% VTDataCAN_4data(3) = fix(CellV_1_104(StrCell*4-1)/4);
% VTDataCAN_4data(4) = fix(CellV_1_104(StrCell*4-0)/4);

Bid = StrCell;
VTDataCAN_64b = uint64( Bid ) + ...
                            uint64( bitshift(uint64(CellV_1_104(StrCell*4-3)/4),8 ) ) + ...
                            uint64( bitshift(uint64(CellV_1_104(StrCell*4-2)/4),8+14 ))  + ...
                            uint64( bitshift(uint64(CellV_1_104(StrCell*4-1)/4),8+14+14)  )  + ...
                            uint64( bitshift(uint64(CellV_1_104(StrCell*4-0)/4),8+14+14+14) ) ;

VTDataCAN_8b(1) = uint8( bitand(VTDataCAN_64b,onemask8_56sft) );
VTDataCAN_8b(2) = uint8( bitand(bitsra(VTDataCAN_64b,8*1),onemask8_56sft) );
VTDataCAN_8b(3) = uint8( bitand(bitsra(VTDataCAN_64b,8*2),onemask8_56sft) );
VTDataCAN_8b(4) = uint8( bitand(bitsra(VTDataCAN_64b,8*3),onemask8_56sft) );
VTDataCAN_8b(5) = uint8( bitand(bitsra(VTDataCAN_64b,8*4),onemask8_56sft) );
VTDataCAN_8b(6) = uint8( bitand(bitsra(VTDataCAN_64b,8*5),onemask8_56sft) );
VTDataCAN_8b(7) = uint8( bitand(bitsra(VTDataCAN_64b,8*6),onemask8_56sft) );
VTDataCAN_8b(8) = uint8( bitand(bitsra(VTDataCAN_64b,8*7),onemask8_56sft) );

% VTDataCAN_8b(1) = Bid;
% VTDataCAN_8b(2) = VTDataCAN_4data(1)/(2^8);
% VTDataCAN_8b(3) = 4*fix(mod(CellV_1_104(StrCell*4-3),2^8)/4);
% VTDataCAN_8b(3) = VTDataCAN_8b(3) + CellV_1_104(StrCell*4-2)/(2^14);
% VTDataCAN_8b(4) = mod(CellV_1_104(StrCell*4-2),2^14) / (2^8);
% VTDataCAN_8b(5) =  * fix(mod(CellV_1_104(StrCell*4-2),2^6));

4*fix(CellV_1_104(StrCell*4-3)/4);


% VTDataCAN_8b(1) =         CellV_1_104(StrCell*4-3)/256;
% VTDataCAN_8b(2) = mod(CellV_1_104(StrCell*4-3),256);
% VTDataCAN_8b(3) =         CellV_1_104(StrCell*4-2)/256;
% VTDataCAN_8b(4) = mod(CellV_1_104(StrCell*4-2),256);
% VTDataCAN_8b(5) =         CellV_1_104(StrCell*4-1)/256;
% VTDataCAN_8b(6) = mod(CellV_1_104(StrCell*4-1),256);
% VTDataCAN_8b(7) =         CellV_1_104(StrCell*4   )/256;
% VTDataCAN_8b(8) = mod(CellV_1_104(StrCell*4   ),256);

% VTDataCAN_8b(1) =         CellV_1_104(1)/256;
% VTDataCAN_8b(2) = mod(CellV_1_104(1),256);
% VTDataCAN_8b(3) =         CellV_1_104(2)/256;
% VTDataCAN_8b(4) = mod(CellV_1_104(2),256);
% VTDataCAN_8b(5) =         CellV_1_104(9)/256;
% VTDataCAN_8b(6) = mod(CellV_1_104(9),256);
% VTDataCAN_8b(7) =         CellV_1_104(10)/256;
% VTDataCAN_8b(8) = mod(CellV_1_104(10),256);

% VTDataCAN_8b(1) =         uint16(30000)/256;
% VTDataCAN_8b(2) = mod(uint16(30000),256);
% VTDataCAN_8b(3) =         uint16(35000)/256;
% VTDataCAN_8b(4) = mod(uint16(35000),256);
% VTDataCAN_8b(5) =         uint16(33000)/256;
% VTDataCAN_8b(6) = mod(uint16(33000),256);
% VTDataCAN_8b(7) =         uint16(20000)/256;
% VTDataCAN_8b(8) = mod(uint16(20000),256);


end








% CellV_1_104(1) = uint16(1);

% SPIDataStore = uint16(zeros(1,21));
% DataFault =  zeros(1,7);
%
% for i=1:7
%   SPIDataStore(i*3-2) = SPIData(i*8-7)+SPIData(i*8-6)*256;
%   SPIDataStore(i*3-1) = SPIData(i*8-5)+SPIData(i*8-4)*256;
%   SPIDataStore(i*3   ) = SPIData(i*8-3)+SPIData(i*8-2)*256;
%   if (PecChk(i*2-1) == SPIData(i*8-1)) && (PecChk(i*2) == SPIData(i*8))
%     DataFault(i) = 1;
%   else
%     DataFault(i) = 0;
%   end
% end



% onemask8 = uint16(hex2dec('00FF'));
% onemask8_8sft = uint16(hex2dec('FF00'));
% onemask88 = uint8(hex2dec('FF'));
% onemask16 = uint16(hex2dec('FFFF'));
%
% % data_test = zeros(1,2);
% remainder = uint16(16);
%
% for i=1:len
%     ii = uint16(i);
% %     data_test(1,i) = data(ii);
% %     address = 2;
%     address = bitand( ...
%         bitxor( ...
%         uint8(bitsra(remainder,7)),data(ii) ), ...
%         onemask88);
%     remainder = bitxor(bitshift(remainder,8,'uint16'),pec15Table(address+1));
% end
% pec15 = uint16(bitand(bitshift(remainder,1,'uint16'),onemask16));
% pec0 = uint8(bitand(pec15,onemask8));
% pec1 = uint8(bitsra(bitand(pec15,onemask8_8sft),8));

== matlab function can_simple_block_bu11143/DataDumpFast1/RawData to StoreData22 ==
  data: StrCell input; CellV_1_104 data_store_memory; VTDataCAN_8b output uint8
function VTDataCAN_8b = fcn(StrCell)
global CellV_1_104;
onemask8 = uint16(hex2dec('00FF'));
onemask8_8sft = uint16(hex2dec('FF00'));
onemask8_56sft = uint64(hex2dec('FF'));
% yl = uint8(bitand(u,onemask8));
% yh = uint8(bitsra(bitand(u,onemask8_8sft),8));
% bitshift(remainder,8)  shift left
% bitsra(remainder,8)  shift right



VTDataCAN_8b =  uint8(zeros(1,8));
VTDataCAN_64b =  uint64(zeros(1,1));
VTDataCAN_4data =  uint8(zeros(1,4));

% VTDataCAN_4data(1) = fix(CellV_1_104(StrCell*4-3)/4);
% VTDataCAN_4data(2) = fix(CellV_1_104(StrCell*4-2)/4);
% VTDataCAN_4data(3) = fix(CellV_1_104(StrCell*4-1)/4);
% VTDataCAN_4data(4) = fix(CellV_1_104(StrCell*4-0)/4);

Bid = StrCell;
VTDataCAN_64b = uint64( Bid ) + ...
                            uint64( bitshift(uint64(CellV_1_104(StrCell*4-3)/4),8 ) ) + ...
                            uint64( bitshift(uint64(CellV_1_104(StrCell*4-2)/4),8+14 ))  + ...
                            uint64( bitshift(uint64(CellV_1_104(StrCell*4-1)/4),8+14+14)  )  + ...
                            uint64( bitshift(uint64(CellV_1_104(StrCell*4-0)/4),8+14+14+14) ) ;

VTDataCAN_8b(1) = uint8( bitand(VTDataCAN_64b,onemask8_56sft) );
VTDataCAN_8b(2) = uint8( bitand(bitsra(VTDataCAN_64b,8*1),onemask8_56sft) );
VTDataCAN_8b(3) = uint8( bitand(bitsra(VTDataCAN_64b,8*2),onemask8_56sft) );
VTDataCAN_8b(4) = uint8( bitand(bitsra(VTDataCAN_64b,8*3),onemask8_56sft) );
VTDataCAN_8b(5) = uint8( bitand(bitsra(VTDataCAN_64b,8*4),onemask8_56sft) );
VTDataCAN_8b(6) = uint8( bitand(bitsra(VTDataCAN_64b,8*5),onemask8_56sft) );
VTDataCAN_8b(7) = uint8( bitand(bitsra(VTDataCAN_64b,8*6),onemask8_56sft) );
VTDataCAN_8b(8) = uint8( bitand(bitsra(VTDataCAN_64b,8*7),onemask8_56sft) );

% VTDataCAN_8b(1) = Bid;
% VTDataCAN_8b(2) = VTDataCAN_4data(1)/(2^8);
% VTDataCAN_8b(3) = 4*fix(mod(CellV_1_104(StrCell*4-3),2^8)/4);
% VTDataCAN_8b(3) = VTDataCAN_8b(3) + CellV_1_104(StrCell*4-2)/(2^14);
% VTDataCAN_8b(4) = mod(CellV_1_104(StrCell*4-2),2^14) / (2^8);
% VTDataCAN_8b(5) =  * fix(mod(CellV_1_104(StrCell*4-2),2^6));

4*fix(CellV_1_104(StrCell*4-3)/4);


% VTDataCAN_8b(1) =         CellV_1_104(StrCell*4-3)/256;
% VTDataCAN_8b(2) = mod(CellV_1_104(StrCell*4-3),256);
% VTDataCAN_8b(3) =         CellV_1_104(StrCell*4-2)/256;
% VTDataCAN_8b(4) = mod(CellV_1_104(StrCell*4-2),256);
% VTDataCAN_8b(5) =         CellV_1_104(StrCell*4-1)/256;
% VTDataCAN_8b(6) = mod(CellV_1_104(StrCell*4-1),256);
% VTDataCAN_8b(7) =         CellV_1_104(StrCell*4   )/256;
% VTDataCAN_8b(8) = mod(CellV_1_104(StrCell*4   ),256);

% VTDataCAN_8b(1) =         CellV_1_104(1)/256;
% VTDataCAN_8b(2) = mod(CellV_1_104(1),256);
% VTDataCAN_8b(3) =         CellV_1_104(2)/256;
% VTDataCAN_8b(4) = mod(CellV_1_104(2),256);
% VTDataCAN_8b(5) =         CellV_1_104(9)/256;
% VTDataCAN_8b(6) = mod(CellV_1_104(9),256);
% VTDataCAN_8b(7) =         CellV_1_104(10)/256;
% VTDataCAN_8b(8) = mod(CellV_1_104(10),256);

% VTDataCAN_8b(1) =         uint16(30000)/256;
% VTDataCAN_8b(2) = mod(uint16(30000),256);
% VTDataCAN_8b(3) =         uint16(35000)/256;
% VTDataCAN_8b(4) = mod(uint16(35000),256);
% VTDataCAN_8b(5) =         uint16(33000)/256;
% VTDataCAN_8b(6) = mod(uint16(33000),256);
% VTDataCAN_8b(7) =         uint16(20000)/256;
% VTDataCAN_8b(8) = mod(uint16(20000),256);


end








% CellV_1_104(1) = uint16(1);

% SPIDataStore = uint16(zeros(1,21));
% DataFault =  zeros(1,7);
%
% for i=1:7
%   SPIDataStore(i*3-2) = SPIData(i*8-7)+SPIData(i*8-6)*256;
%   SPIDataStore(i*3-1) = SPIData(i*8-5)+SPIData(i*8-4)*256;
%   SPIDataStore(i*3   ) = SPIData(i*8-3)+SPIData(i*8-2)*256;
%   if (PecChk(i*2-1) == SPIData(i*8-1)) && (PecChk(i*2) == SPIData(i*8))
%     DataFault(i) = 1;
%   else
%     DataFault(i) = 0;
%   end
% end



% onemask8 = uint16(hex2dec('00FF'));
% onemask8_8sft = uint16(hex2dec('FF00'));
% onemask88 = uint8(hex2dec('FF'));
% onemask16 = uint16(hex2dec('FFFF'));
%
% % data_test = zeros(1,2);
% remainder = uint16(16);
%
% for i=1:len
%     ii = uint16(i);
% %     data_test(1,i) = data(ii);
% %     address = 2;
%     address = bitand( ...
%         bitxor( ...
%         uint8(bitsra(remainder,7)),data(ii) ), ...
%         onemask88);
%     remainder = bitxor(bitshift(remainder,8,'uint16'),pec15Table(address+1));
% end
% pec15 = uint16(bitand(bitshift(remainder,1,'uint16'),onemask16));
% pec0 = uint8(bitand(pec15,onemask8));
% pec1 = uint8(bitsra(bitand(pec15,onemask8_8sft),8));

== matlab function can_simple_block_bu11143/DataDumpFast1/RawData to StoreData23 ==
  data: StrCell input; CellV_1_104 data_store_memory; VTDataCAN_8b output uint8
function VTDataCAN_8b = fcn(StrCell)
global CellV_1_104;
onemask8 = uint16(hex2dec('00FF'));
onemask8_8sft = uint16(hex2dec('FF00'));
onemask8_56sft = uint64(hex2dec('FF'));
% yl = uint8(bitand(u,onemask8));
% yh = uint8(bitsra(bitand(u,onemask8_8sft),8));
% bitshift(remainder,8)  shift left
% bitsra(remainder,8)  shift right



VTDataCAN_8b =  uint8(zeros(1,8));
VTDataCAN_64b =  uint64(zeros(1,1));
VTDataCAN_4data =  uint8(zeros(1,4));

% VTDataCAN_4data(1) = fix(CellV_1_104(StrCell*4-3)/4);
% VTDataCAN_4data(2) = fix(CellV_1_104(StrCell*4-2)/4);
% VTDataCAN_4data(3) = fix(CellV_1_104(StrCell*4-1)/4);
% VTDataCAN_4data(4) = fix(CellV_1_104(StrCell*4-0)/4);

Bid = StrCell;
VTDataCAN_64b = uint64( Bid ) + ...
                            uint64( bitshift(uint64(CellV_1_104(StrCell*4-3)/4),8 ) ) + ...
                            uint64( bitshift(uint64(CellV_1_104(StrCell*4-2)/4),8+14 ))  + ...
                            uint64( bitshift(uint64(CellV_1_104(StrCell*4-1)/4),8+14+14)  )  + ...
                            uint64( bitshift(uint64(CellV_1_104(StrCell*4-0)/4),8+14+14+14) ) ;

VTDataCAN_8b(1) = uint8( bitand(VTDataCAN_64b,onemask8_56sft) );
VTDataCAN_8b(2) = uint8( bitand(bitsra(VTDataCAN_64b,8*1),onemask8_56sft) );
VTDataCAN_8b(3) = uint8( bitand(bitsra(VTDataCAN_64b,8*2),onemask8_56sft) );
VTDataCAN_8b(4) = uint8( bitand(bitsra(VTDataCAN_64b,8*3),onemask8_56sft) );
VTDataCAN_8b(5) = uint8( bitand(bitsra(VTDataCAN_64b,8*4),onemask8_56sft) );
VTDataCAN_8b(6) = uint8( bitand(bitsra(VTDataCAN_64b,8*5),onemask8_56sft) );
VTDataCAN_8b(7) = uint8( bitand(bitsra(VTDataCAN_64b,8*6),onemask8_56sft) );
VTDataCAN_8b(8) = uint8( bitand(bitsra(VTDataCAN_64b,8*7),onemask8_56sft) );

% VTDataCAN_8b(1) = Bid;
% VTDataCAN_8b(2) = VTDataCAN_4data(1)/(2^8);
% VTDataCAN_8b(3) = 4*fix(mod(CellV_1_104(StrCell*4-3),2^8)/4);
% VTDataCAN_8b(3) = VTDataCAN_8b(3) + CellV_1_104(StrCell*4-2)/(2^14);
% VTDataCAN_8b(4) = mod(CellV_1_104(StrCell*4-2),2^14) / (2^8);
% VTDataCAN_8b(5) =  * fix(mod(CellV_1_104(StrCell*4-2),2^6));

4*fix(CellV_1_104(StrCell*4-3)/4);


% VTDataCAN_8b(1) =         CellV_1_104(StrCell*4-3)/256;
% VTDataCAN_8b(2) = mod(CellV_1_104(StrCell*4-3),256);
% VTDataCAN_8b(3) =         CellV_1_104(StrCell*4-2)/256;
% VTDataCAN_8b(4) = mod(CellV_1_104(StrCell*4-2),256);
% VTDataCAN_8b(5) =         CellV_1_104(StrCell*4-1)/256;
% VTDataCAN_8b(6) = mod(CellV_1_104(StrCell*4-1),256);
% VTDataCAN_8b(7) =         CellV_1_104(StrCell*4   )/256;
% VTDataCAN_8b(8) = mod(CellV_1_104(StrCell*4   ),256);

% VTDataCAN_8b(1) =         CellV_1_104(1)/256;
% VTDataCAN_8b(2) = mod(CellV_1_104(1),256);
% VTDataCAN_8b(3) =         CellV_1_104(2)/256;
% VTDataCAN_8b(4) = mod(CellV_1_104(2),256);
% VTDataCAN_8b(5) =         CellV_1_104(9)/256;
% VTDataCAN_8b(6) = mod(CellV_1_104(9),256);
% VTDataCAN_8b(7) =         CellV_1_104(10)/256;
% VTDataCAN_8b(8) = mod(CellV_1_104(10),256);

% VTDataCAN_8b(1) =         uint16(30000)/256;
% VTDataCAN_8b(2) = mod(uint16(30000),256);
% VTDataCAN_8b(3) =         uint16(35000)/256;
% VTDataCAN_8b(4) = mod(uint16(35000),256);
% VTDataCAN_8b(5) =         uint16(33000)/256;
% VTDataCAN_8b(6) = mod(uint16(33000),256);
% VTDataCAN_8b(7) =         uint16(20000)/256;
% VTDataCAN_8b(8) = mod(uint16(20000),256);


end








% CellV_1_104(1) = uint16(1);

% SPIDataStore = uint16(zeros(1,21));
% DataFault =  zeros(1,7);
%
% for i=1:7
%   SPIDataStore(i*3-2) = SPIData(i*8-7)+SPIData(i*8-6)*256;
%   SPIDataStore(i*3-1) = SPIData(i*8-5)+SPIData(i*8-4)*256;
%   SPIDataStore(i*3   ) = SPIData(i*8-3)+SPIData(i*8-2)*256;
%   if (PecChk(i*2-1) == SPIData(i*8-1)) && (PecChk(i*2) == SPIData(i*8))
%     DataFault(i) = 1;
%   else
%     DataFault(i) = 0;
%   end
% end



% onemask8 = uint16(hex2dec('00FF'));
% onemask8_8sft = uint16(hex2dec('FF00'));
% onemask88 = uint8(hex2dec('FF'));
% onemask16 = uint16(hex2dec('FFFF'));
%
% % data_test = zeros(1,2);
% remainder = uint16(16);
%
% for i=1:len
%     ii = uint16(i);
% %     data_test(1,i) = data(ii);
% %     address = 2;
%     address = bitand( ...
%         bitxor( ...
%         uint8(bitsra(remainder,7)),data(ii) ), ...
%         onemask88);
%     remainder = bitxor(bitshift(remainder,8,'uint16'),pec15Table(address+1));
% end
% pec15 = uint16(bitand(bitshift(remainder,1,'uint16'),onemask16));
% pec0 = uint8(bitand(pec15,onemask8));
% pec1 = uint8(bitsra(bitand(pec15,onemask8_8sft),8));
